simulink model "simulink_3"  (R2020a)
settings: Solver=VariableStepAuto  StartTime=0.0  StopTime=10.0  RelTol=1e-3
settings Model: Creator=joshi  LastModifiedBy=joshi

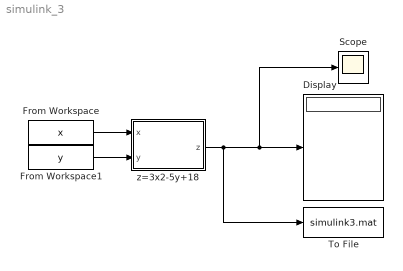
== system simulink_3 ==
  Display : Display
  From Workspace : FromWorkspace  VariableName=x
  From Workspace1 : FromWorkspace  VariableName=y
  Scope : Scope
  To File : ToFile  Filename=simulink3.mat  MatrixName=function_output  SaveFormat=Timeseries
  z=3x2-5y+18 : MATLAB Function  TreatAsAtomicUnit=on
  wires:
  From Workspace1/1 -> z=3x2-5y+18/2(y)
  From Workspace/1 -> z=3x2-5y+18/1(x)
  z=3x2-5y+18/1(z) -> Scope/1, Display/1, To File/1

== matlab function simulink_3/z=3x2-5y+18 ==
  data: x input; z output; y input
function z  = fcn(x,y)

[z] = 3*x.*x-5.*y +18 ;
end
